simulink model "EPD629_WilliamsJ_AS04_P3_simulink"  (R2021b)
settings: Solver=VariableStepAuto  StartTime=0.0  StopTime=1  RelTol=1e-3
values from neighbouring files (symbols this model uses):
  b = 0.001    [EPD629_WilliamsJ_AS04.m]
  J = 50e-6    (= 5e-05)    [EPD629_WilliamsJ_AS04.m]
  MotorTorque = 1    [EPD629_WilliamsJ_AS04.m]
undefined symbols (not defined in the file or in its folder): A2, B2, C2, D2
settings Model: Creator=jwilli42  LastModifiedBy=jwilli42

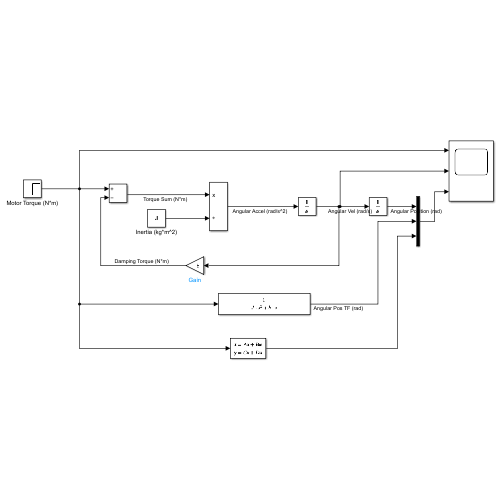
[thumbnail: Simulink's stored preview of the top-level diagram]
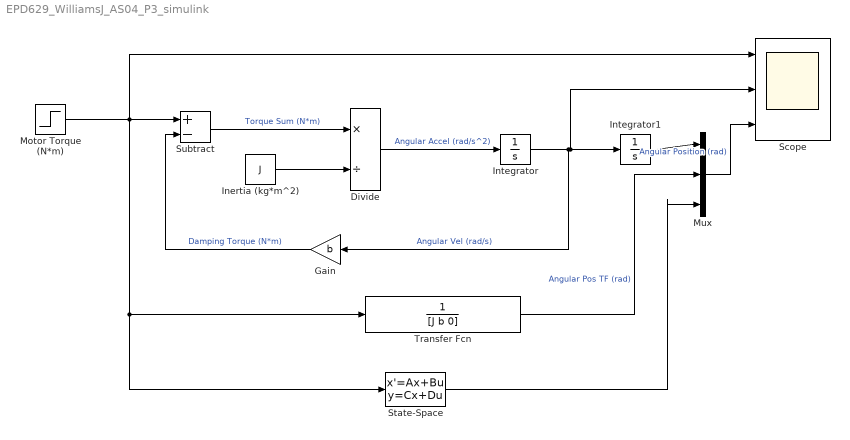
== system EPD629_WilliamsJ_AS04_P3_simulink ==
  Divide : Product  Inputs=*/
  Gain : Gain  Gain=b
  Inertia (kg*m^2) : Constant  Value=J
  Integrator : Integrator
  Integrator1 : Integrator
  Motor Torque (N*m) : Step  Time=0  After=MotorTorque  SampleTime=0
  Mux : Mux  Inputs=3
  Scope : Scope  NumInputPorts=3
  State-Space : StateSpace  A=A2  B=B2  C=C2  D=D2  InitialCondition=0
  Subtract : Sum  Inputs=+-
  Transfer Fcn : TransferFcn  Denominator=[J b 0]
  wires:
  Motor Torque (N*m)/1 -> State-Space/1, Transfer Fcn/1, Scope/1, Subtract/1
  Subtract/1 -> Divide/1  "Torque Sum (N*m)"
  Divide/1 -> Integrator/1  "Angular Accel (rad/s^2)"
  Integrator/1 -> Scope/2, Integrator1/1, Gain/1  "Angular Vel (rad/s)"
  Inertia (kg*m^2)/1 -> Divide/2
  Gain/1 -> Subtract/2  "Damping Torque (N*m)"
  Mux/1 -> Scope/3
  Transfer Fcn/1 -> Mux/2  "Angular Pos TF (rad)"
  State-Space/1 -> Mux/3
  Integrator1/1 -> Mux/1  "Angular Position (rad)"
